simulink model "q2section2"  (R2019a)
settings: Solver=VariableStepAuto  StartTime=0.0  StopTime=6  RelTol=1e-3
values from neighbouring files (symbols this model uses):
  g = 9.81    [q2.m]
  mL = 1000    [q2.m]
libraries: cstblocks x2
settings Model: Creator=Nir Lalum  LastModifiedBy=Nir Lalum

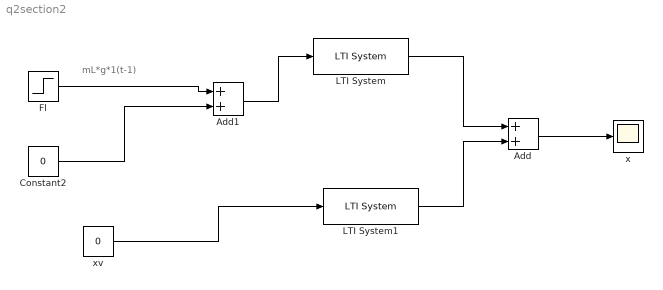
== system q2section2 ==
  note: mL*g*1(t-1)
  Add : Sum
  Add1 : Sum
  Constant2 : Constant  Value=0
  Fl : Step  Before=mL*g  After=0  SampleTime=0
  LTI System : cstblocks/LTI System  sys=Pf  IC=[]
  LTI System1 : cstblocks/LTI System  sys=Pxv  IC=[]
  "x " : Scope
  xv : Constant  Value=0
  wires:
  xv/1 -> LTI System1/1
  LTI System/1 -> Add/1
  LTI System1/1 -> Add/2
  Add/1 -> "x "/1
  Fl/1 -> Add1/1
  Constant2/1 -> Add1/2
  Add1/1 -> LTI System/1
